simulink model "resultsTesting"  (R2019a)
settings: Solver=VariableStepAuto  StartTime=0.0  StopTime=50  RelTol=1e-3
values from neighbouring files (symbols this model uses):
  Kp_1 = b/a    [pcAssign1.m]
  Kp_2 = bw    [pcAssign1.m]
  Kp_3 = Kp_2    [pcAssign1.m]
  L_1 = theta(2,1)/theta(3,1)    [pcAssign1.m]
  L_2 = Lw/Num2    (= 0)    [pcAssign1.m]
  L_3 = data(i,3)    [pcAssign1.m]
  Ts_1 = 1/a    [pcAssign1.m]
  Ts_2 = aw    [pcAssign1.m]
  Ts_3 = sqrt((Kp_3*Ku_3)^2-1)/wu_3    [pcAssign1.m]
settings Model: Creator=Administrator  LastModifiedBy=Administrator

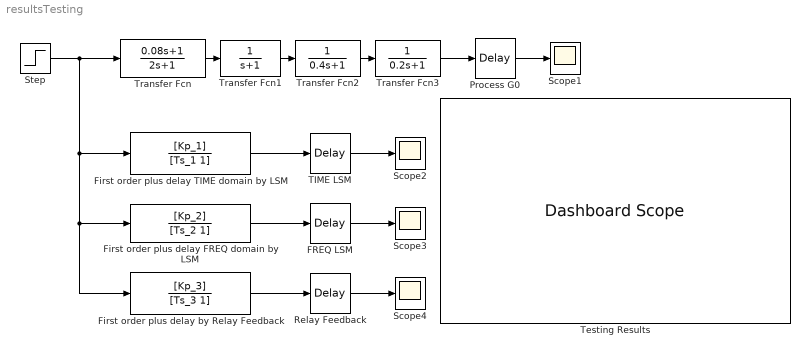
== system resultsTesting ==
  FREQ LSM : TransportDelay  DelayTime=L_2
  First order plus delay FREQ domain by LSM : TransferFcn  Numerator=[Kp_2]  Denominator=[Ts_2 1]  AbsoluteTolerance=1
  First order plus delay TIME domain by LSM : TransferFcn  Numerator=[Kp_1]  Denominator=[Ts_1 1]  AbsoluteTolerance=1
  First order plus delay by Relay Feedback : TransferFcn  Numerator=[Kp_3]  Denominator=[Ts_3 1]  AbsoluteTolerance=1
  Process G0 : TransportDelay  DelayTime=3
  Relay Feedback : TransportDelay  DelayTime=L_3
  Scope{1..4} (4 alike) : Scope
  Step : Step  SampleTime=0
  TIME LSM : TransportDelay  DelayTime=L_1
  Testing Results : DashboardScope
  Transfer Fcn : TransferFcn  Numerator=[0.08 1]  Denominator=[2 1]
  Transfer Fcn1 : TransferFcn  Denominator=[1 1]
  Transfer Fcn2 : TransferFcn  Denominator=[0.4 1]
  Transfer Fcn3 : TransferFcn  Denominator=[0.2 1]
  wires:
  Transfer Fcn/1 -> Transfer Fcn1/1
  Transfer Fcn3/1 -> Process G0/1
  Transfer Fcn2/1 -> Transfer Fcn3/1
  Transfer Fcn1/1 -> Transfer Fcn2/1
  Process G0/1 -> Scope1/1
  TIME LSM/1 -> Scope2/1
  Step/1 -> First order plus delay by Relay Feedback/1, First order plus delay FREQ domain by LSM/1, First order plus delay TIME domain by LSM/1, Transfer Fcn/1
  First order plus delay TIME domain by LSM/1 -> TIME LSM/1
  First order plus delay FREQ domain by LSM/1 -> FREQ LSM/1
  FREQ LSM/1 -> Scope3/1
  Relay Feedback/1 -> Scope4/1
  First order plus delay by Relay Feedback/1 -> Relay Feedback/1
